simulink library "lddc_lib"  (Simulink 8.7)
settings: Solver=ode45  StartTime=0.0  StopTime=10.0  RelTol=1e-3
undefined symbols (not defined in the file): DDC_LINEUP_param, display, value
libraries: DSPBAPrim x9, DSPBAFilters x6, DSPBABase x6
settings Model: Creator=bigcat  LastModifiedBy=5g

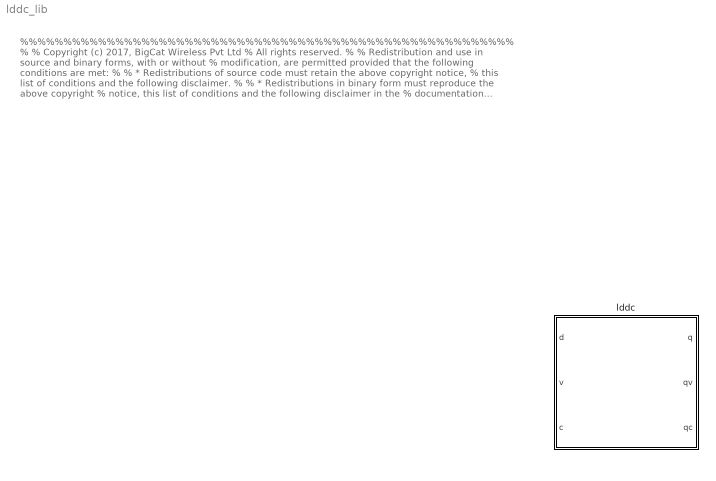
== system lddc_lib ==
  note: %%%%%%%%%%%%%%%%%%%%%%%%%%%%%%%%%%%%%%%%%%%%%%%%%%%%%%%%%
      |  %
      |  % Copyright (c) 2017, BigCat Wireless Pvt Ltd
      |  % All rights reserved.
      |  %
      |  % Redistribution and use in source and binary forms, with or without
      |  % modification, are permitted provided that the following conditions are met:
      |  %
      |  %     * Redistributions of source code must retain the above copyright notice,
      |  %       this list of conditions and the following disclaimer.
      |  %
      |  %     * Redistributions in binary form must reproduce the above copyright
      |  %       notice, this list of conditions and the following disclaimer in the
      |  %       documentation and/or other materials provided with the distribution.
      |  %
      |  %     * Neither the name of the copyright holder nor the names of its contributors
      |  %       may be used to endorse or promote products derived from this software
      |  %       without specific prior written permission.
      |  %
      |  %
      |  %
      |  % THIS SOFTWARE IS PROVIDED BY THE COPYRIGHT HOLDERS AND CONTRIBUTORS "AS IS"
      |  % AND ANY EXPRESS OR IMPLIED WARRANTIES, INCLUDING, BUT NOT LIMITED TO, THE
      |  % IMPLIED WARRANTIES OF MERCHANTABILITY AND FITNESS FOR A PARTICULAR PURPOSE ARE
      |  % DISCLAIMED. IN NO EVENT SHALL THE COPYRIGHT HOLDER OR CONTRIBUTORS BE LIABLE
      |  % FOR ANY DIRECT, INDIRECT, INCIDENTAL, SPECIAL, EXEMPLARY, OR CONSEQUENTIAL
      |  % DAMAGES (INCLUDING, BUT NOT LIMITED TO, PROCUREMENT OF SUBSTITUTE GOODS OR
      |  % SERVICES; LOSS OF USE, DATA, OR PROFITS; OR BUSINESS INTERRUPTION) HOWEVER
      |  % CAUSED AND ON ANY THEORY OF LIABILITY, WHETHER IN CONTRACT, STRICT LIABILITY,
      |  % OR TORT (INCLUDING NEGLIGENCE OR OTHERWISE) ARISING IN ANY WAY OUT OF THE USE
      |  % OF THIS SOFTWARE, EVEN IF ADVISED OF THE POSSIBILITY OF SUCH DAMAGE.
      |  %
      |   %%%%%%%%%%%%%%%%%%%%%%%%%%%%%%%%%%%%%%%%%%%%%%%%%%%%%
  lddc : Subsystem  mask{HB5_filter_SampleRate=DDC_LINEUP_param.HB_filter5.SampleRate, HB5_filter_Decimation=DDC_LINEUP_param.HB_filter5.Decimation, HB5_filter_ChanCount=DDC_LINEUP_param.HB_filter5.ChanCount, HB5_filter_coeffs=DDC_LINEUP_param.HB_filt5.coeffs(1,:), HB5_filter_base_addr=DDC_LINEUP_param.HB_filter5.base_addr, HB4_filter_SampleRate=DDC_LINEUP_param.HB_filter4.SampleRate, HB4_filter_Decimation=DDC_LINEUP_param.HB_filter4.Decimation, HB4_filter_ChanCount=DDC_LINEUP_param.HB_filter4.ChanCount, HB4_filter_coeffs=DDC_LINEUP_param.HB_filt4.coeffs(1,:), HB4_filter_base_addr=DDC_LINEUP_param.HB_filter4.base_addr, CH_filter_SampleRate=DDC_LINEUP_param.CH_filter.SampleRate, CH_filter_ChanCount=DDC_LINEUP_param.CH_filter.ChanCount, CH_filter_coeffs=DDC_LINEUP_param.chan_filter.coeffs(1,:), CH_filter_base_addr=DDC_LINEUP_param.CH_filter.base_addr, output_word_length=DDC_LINEUP_param.output_word_length, output_fraction_length=DDC_LINEUP_param.output_fraction_length, Pipeline_stages=2, Clock_Margin=DDC_LINEUP_param.ClockMargin}
      mask Display:
      | disp('LDDC');
      | port_label('input',1,'d');
      | port_label('input',2,'v');
      | port_label('input',3,'c');
      | port_label('output',1,'q');
      | port_label('output',2,'q_v');
      | port_label('output',3,'q_c');

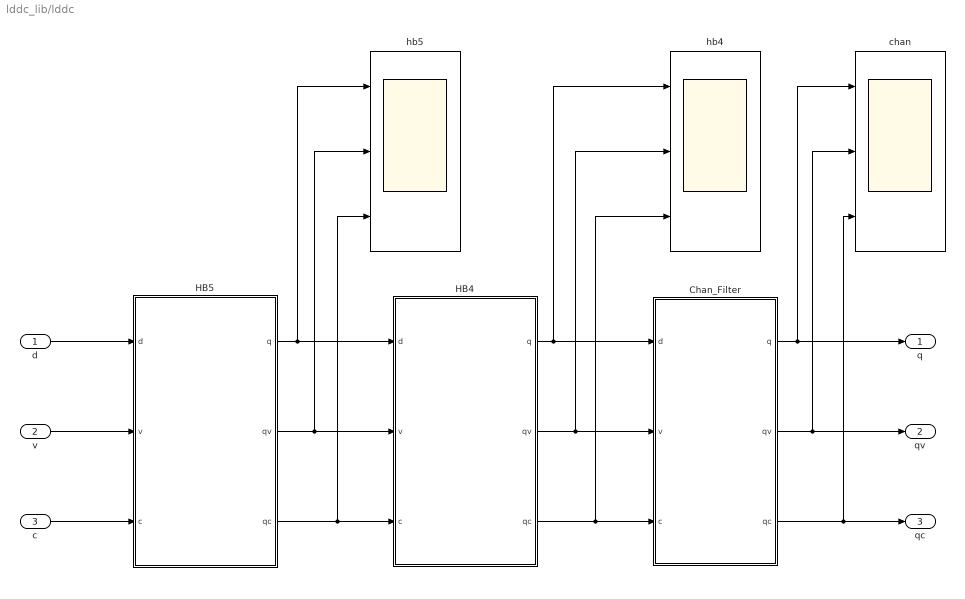
== system lddc_lib/lddc ==
  d : Inport
  v : Inport  Port=2
  c : Inport  Port=3
  Chan_Filter : Subsystem
  HB4 : Subsystem
  HB5 : Subsystem
  chan : Scope  NumInputPorts=3
  hb4 : Scope  NumInputPorts=3
  hb5 : Scope  NumInputPorts=3
  q : Outport
  qv : Outport  Port=2
  qc : Outport  Port=3
  wires:
  HB4/3(qc) -> hb4/3, Chan_Filter/3(c)
  HB4/2(qv) -> hb4/2, Chan_Filter/2(v)
  HB4/1(q) -> hb4/1, Chan_Filter/1(d)
  HB5/3(qc) -> hb5/3, HB4/3(c)
  HB5/2(qv) -> hb5/2, HB4/2(v)
  HB5/1(q) -> hb5/1, HB4/1(d)
  d/1 -> HB5/1(d)
  v/1 -> HB5/2(v)
  c/1 -> HB5/3(c)
  Chan_Filter/1(q) -> chan/1, q/1
  Chan_Filter/2(qv) -> chan/2, qv/1
  Chan_Filter/3(qc) -> chan/3, qc/1

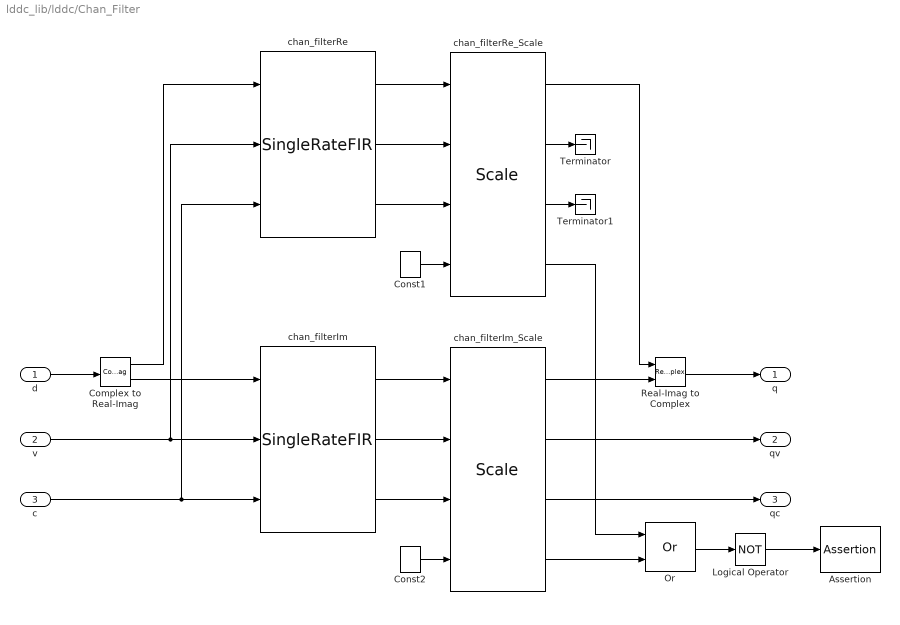
== system lddc_lib/lddc/Chan_Filter ==
  d : Inport
  v : Inport  Port=2
  c : Inport  Port=3
  Assertion : Assertion  Enabled=off  AssertionFailFcn=display('Simulation stopped, because an over/underflow was detected in LDDC/HB5')
  Complex to Real-Imag : ComplexToRealImag
  Const1 : DSPBAPrim/Const  primtype=const  nInputs=0  nOutputs=1  omode=Inherit via internal rule  otype=sfix(16)  scale=2^-15  rndmethod=Unbiased  factor=1  satmethod=Symmetric  shift_vec=[0 1 2 -1]  value=0  inPortNames=['+'; '+';]  outPortNames=[' ']  dspbaimage=dspba_prim.jpg  text=fprintf('%s', num2str(value));  style=Optimised  visibilities=8 + 1024  floatPrecision=float32_m23  version=20120820
  Const2 : DSPBAPrim/Const  primtype=const  nInputs=0  nOutputs=1  omode=Inherit via internal rule  otype=sfix(16)  scale=2^-15  rndmethod=Unbiased  factor=1  satmethod=Symmetric  shift_vec=[0 1 2 -1]  value=0  inPortNames=['+'; '+';]  outPortNames=[' ']  dspbaimage=dspba_prim.jpg  text=fprintf('%s', num2str(value));  style=Optimised  visibilities=8 + 1024  floatPrecision=float32_m23  version=20120820
  Logical Operator : Logic  Operator=NOT  AllPortsSameDT=off  OutDataTypeStr=boolean
  Or : DSPBAPrim/Or  primtype=or  nInputs=2  nOutputs=1  omode=Inherit via internal rule  otype=sfix(16)  scale=2^-15  rndmethod=Unbiased  factor=1  satmethod=Symmetric  shift_vec=[0 1 2 -1]  value=0  inPortNames=[' '; ' '; ' '; ' '; ' '; ' '; ' '; ' '; ' '; ' '; ' '; ' '; ' '; ' '; ' '; ' '; ]  outPortNames=[' ']  dspbaimage=dspba_prim.jpg  text=fprintf('|');  style=Optimised  visibilities=8+2  version=20090407
  Real-Imag to Complex : RealImagToComplex
  Terminator : Terminator
  Terminator1 : Terminator
  chan_filterIm : DSPBAFilters/SingleRateFIR  nInputRate=CH_filter_SampleRate  nchan=CH_filter_ChanCount  symmetry=Symmetrical  coef=fi(CH_filter_coeffs,1,16,15)  addr=CH_filter_base_addr+64  rwmode=Read/Write  nband=Use All Taps  latency=4  exposebus=off  version=20090407  recon=off  MM=[0,1,2,3,4,5,6,7,8,9,10,11,12,13,14,15,16,17,18,19]
  chan_filterIm_Scale : DSPBABase/Scale  otype=sfix(output_word_length)  scale=2^-output_fraction_length  rndmethod=Truncate  factor=1  satmethod=Symmetric  shift_vec=0  latency=4  wideSimulation=off  version=20130807
  chan_filterRe : DSPBAFilters/SingleRateFIR  nInputRate=CH_filter_SampleRate  nchan=CH_filter_ChanCount  symmetry=Symmetrical  coef=fi(CH_filter_coeffs,1,16,15)  addr=CH_filter_base_addr  rwmode=Read/Write  nband=Use All Taps  latency=4  exposebus=off  version=20090407  recon=off  MM=[0,1,2,3,4,5,6,7,8,9,10,11,12,13,14,15,16,17,18,19]
  chan_filterRe_Scale : DSPBABase/Scale  otype=sfix(output_word_length)  scale=2^-output_fraction_length  rndmethod=Truncate  factor=1  satmethod=Symmetric  shift_vec=0  latency=4  wideSimulation=off  version=20130807
  q : Outport
  qv : Outport  Port=2
  qc : Outport  Port=3
  wires:
  v/1 -> chan_filterIm/2, chan_filterRe/2
  Or/1 -> Logical Operator/1
  Logical Operator/1 -> Assertion/1
  Real-Imag to Complex/1 -> q/1
  chan_filterIm_Scale/1 -> Real-Imag to Complex/2
  chan_filterRe_Scale/1 -> Real-Imag to Complex/1
  chan_filterRe_Scale/4 -> Or/1
  chan_filterIm_Scale/4 -> Or/2
  Complex to Real-Imag/1 -> chan_filterRe/1
  Complex to Real-Imag/2 -> chan_filterIm/1
  d/1 -> Complex to Real-Imag/1
  chan_filterRe/2 -> chan_filterRe_Scale/2
  chan_filterRe/3 -> chan_filterRe_Scale/3
  Const1/1 -> chan_filterRe_Scale/4
  chan_filterRe/1 -> chan_filterRe_Scale/1
  chan_filterIm/2 -> chan_filterIm_Scale/2
  chan_filterIm/3 -> chan_filterIm_Scale/3
  chan_filterIm_Scale/2 -> qv/1
  Const2/1 -> chan_filterIm_Scale/4
  chan_filterIm_Scale/3 -> qc/1
  chan_filterIm/1 -> chan_filterIm_Scale/1
  c/1 -> chan_filterIm/3, chan_filterRe/3
  chan_filterRe_Scale/2 -> Terminator/1
  chan_filterRe_Scale/3 -> Terminator1/1

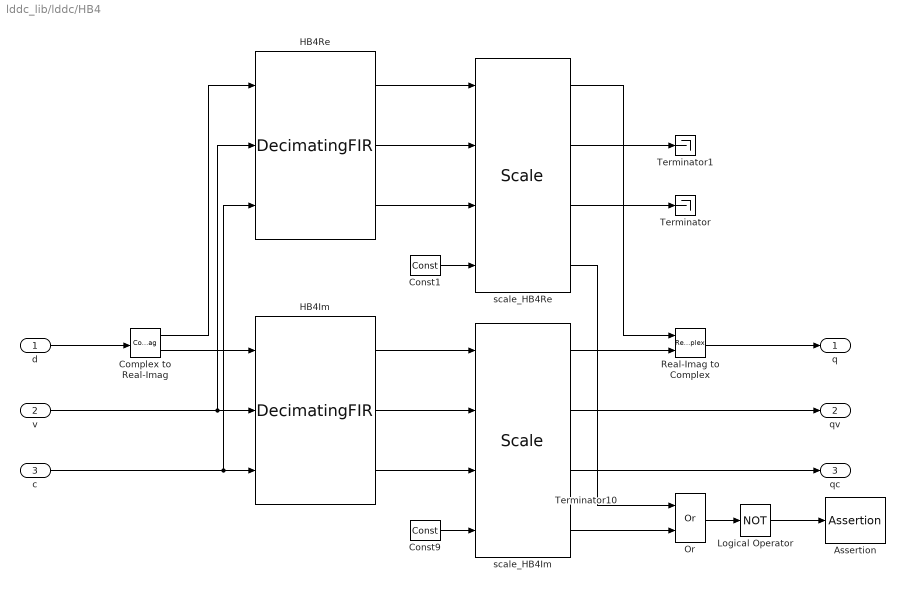
== system lddc_lib/lddc/HB4 ==
  d : Inport
  v : Inport  Port=2
  c : Inport  Port=3
  Assertion : Assertion  Enabled=off  AssertionFailFcn=display('Simulation stopped, because an over/underflow was detected in LDDC/HB4')
  Complex to Real-Imag : ComplexToRealImag
  Const1 : DSPBAPrim/Const  primtype=const  nInputs=0  nOutputs=1  omode=Inherit via internal rule  otype=sfix(16)  scale=2^-15  rndmethod=Unbiased  factor=1  satmethod=Symmetric  shift_vec=[0 1 2 -1]  value=0  inPortNames=['+'; '+';]  outPortNames=[' ']  dspbaimage=dspba_prim.jpg  text=fprintf('%s', num2str(value));  style=Optimised  visibilities=8 + 1024  floatPrecision=float32_m23  version=20120820
  Const9 : DSPBAPrim/Const  primtype=const  nInputs=0  nOutputs=1  omode=Inherit via internal rule  otype=sfix(16)  scale=2^-15  rndmethod=Unbiased  factor=1  satmethod=Symmetric  shift_vec=[0 1 2 -1]  value=0  inPortNames=['+'; '+';]  outPortNames=[' ']  dspbaimage=dspba_prim.jpg  text=fprintf('%s', num2str(value));  style=Optimised  visibilities=8 + 1024  floatPrecision=float32_m23  version=20120820
  HB4Im : DSPBAFilters/DecimatingFIR  nInputRate=HB4_filter_SampleRate  decim=HB4_filter_Decimation  nchan=HB4_filter_ChanCount  symmetry=Symmetrical  coef=HB4_filter_coeffs  addr=HB4_filter_base_addr  rwmode=Constant  nband=Half Band  exposebus=off  latency=23  version=20090407  recon=off  MM=[0,1,2,3,4,5,6,7,8,9,10,11,12,13,14,15]
  HB4Re : DSPBAFilters/DecimatingFIR  nInputRate=HB4_filter_SampleRate  decim=HB4_filter_Decimation  nchan=HB4_filter_ChanCount  symmetry=Symmetrical  coef=HB4_filter_coeffs  addr=HB4_filter_base_addr  rwmode=Constant  nband=Half Band  exposebus=off  latency=23  version=20090407  recon=off  MM=[0,1,2,3,4,5,6,7,8,9,10,11,12,13,14,15]
  Logical Operator : Logic  Operator=NOT  AllPortsSameDT=off  OutDataTypeStr=boolean
  Or : DSPBAPrim/Or  primtype=or  nInputs=2  nOutputs=1  omode=Inherit via internal rule  otype=sfix(16)  scale=2^-15  rndmethod=Unbiased  factor=1  satmethod=Symmetric  shift_vec=[0 1 2 -1]  value=0  inPortNames=[' '; ' '; ' '; ' '; ' '; ' '; ' '; ' '; ' '; ' '; ' '; ' '; ' '; ' '; ' '; ' '; ]  outPortNames=[' ']  dspbaimage=dspba_prim.jpg  text=fprintf('|');  style=Optimised  visibilities=8+2  version=20090407
  Real-Imag to Complex : RealImagToComplex
  Terminator : Terminator
  Terminator1 : Terminator
  Terminator10 : Terminator
  scale_HB4Im : DSPBABase/Scale  otype=sfix(output_word_length)  scale=2^-output_fraction_length  rndmethod=Truncate  factor=1  satmethod=Symmetric  shift_vec=0  latency=4  wideSimulation=off  version=20130807
  scale_HB4Re : DSPBABase/Scale  otype=sfix(output_word_length)  scale=2^-output_fraction_length  rndmethod=Truncate  factor=1  satmethod=Symmetric  shift_vec=0  latency=4  wideSimulation=off  version=20130807
  q : Outport
  qv : Outport  Port=2
  qc : Outport  Port=3
  wires:
  v/1 -> HB4Im/2, HB4Re/2
  Or/1 -> Logical Operator/1
  Logical Operator/1 -> Assertion/1
  scale_HB4Im/1 -> Real-Imag to Complex/2
  scale_HB4Re/4 -> Or/1
  scale_HB4Re/1 -> Real-Imag to Complex/1
  Complex to Real-Imag/2 -> HB4Im/1
  Complex to Real-Imag/1 -> HB4Re/1
  Real-Imag to Complex/1 -> q/1
  scale_HB4Im/4 -> Or/2
  d/1 -> Complex to Real-Imag/1
  HB4Re/3 -> scale_HB4Re/3
  HB4Re/1 -> scale_HB4Re/1
  HB4Re/2 -> scale_HB4Re/2
  Const1/1 -> scale_HB4Re/4
  HB4Im/3 -> scale_HB4Im/3
  HB4Im/1 -> scale_HB4Im/1
  HB4Im/2 -> scale_HB4Im/2
  Const9/1 -> scale_HB4Im/4
  c/1 -> HB4Im/3, HB4Re/3
  scale_HB4Im/3 -> qc/1
  scale_HB4Im/2 -> qv/1
  scale_HB4Re/3 -> Terminator/1
  scale_HB4Re/2 -> Terminator1/1

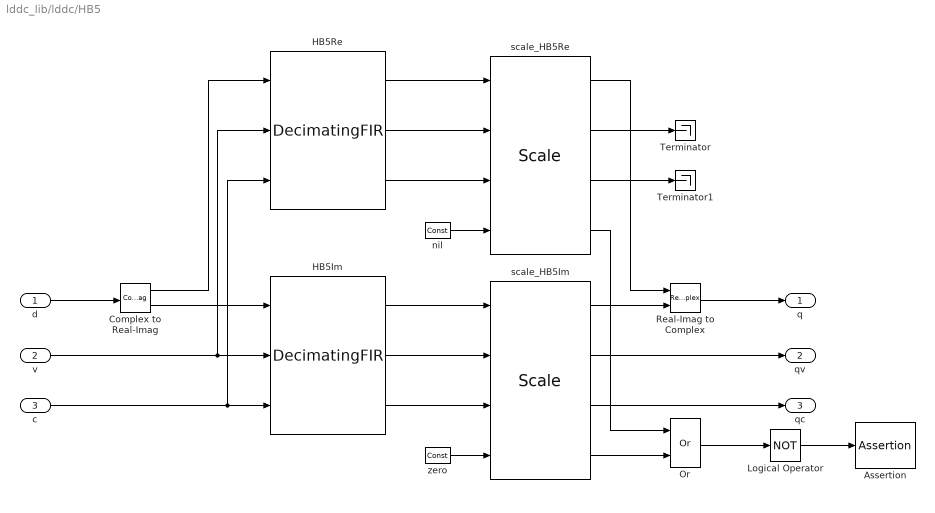
== system lddc_lib/lddc/HB5 ==
  d : Inport
  v : Inport  Port=2
  c : Inport  Port=3
  Assertion : Assertion  Enabled=off  AssertionFailFcn=display('Simulation stopped, because an over/underflow was detected in LDDC/HB5')
  Complex to Real-Imag : ComplexToRealImag
  HB5Im : DSPBAFilters/DecimatingFIR  nInputRate=HB5_filter_SampleRate  decim=HB5_filter_Decimation  nchan=HB5_filter_ChanCount  symmetry=Symmetrical  coef=HB5_filter_coeffs  addr=HB5_filter_base_addr  rwmode=Constant  nband=Half Band  exposebus=off  latency=19  version=20090407  recon=off  MM=[0,1,2,3,4,5,6,7,8,9,10,11,12,13,14,15]
  HB5Re : DSPBAFilters/DecimatingFIR  nInputRate=HB5_filter_SampleRate  decim=HB5_filter_Decimation  nchan=HB5_filter_ChanCount  symmetry=Symmetrical  coef=HB5_filter_coeffs  addr=HB5_filter_base_addr  rwmode=Constant  nband=Half Band  exposebus=off  latency=19  version=20090407  recon=off  MM=[0,1,2,3,4,5,6,7,8,9,10,11,12,13,14,15]
  Logical Operator : Logic  Operator=NOT  AllPortsSameDT=off  OutDataTypeStr=boolean
  Or : DSPBAPrim/Or  primtype=or  nInputs=2  nOutputs=1  omode=Inherit via internal rule  otype=sfix(16)  scale=2^-15  rndmethod=Unbiased  factor=1  satmethod=Symmetric  shift_vec=[0 1 2 -1]  value=0  inPortNames=[' '; ' '; ' '; ' '; ' '; ' '; ' '; ' '; ' '; ' '; ' '; ' '; ' '; ' '; ' '; ' '; ]  outPortNames=[' ']  dspbaimage=dspba_prim.jpg  text=fprintf('|');  style=Optimised  visibilities=8+2  version=20090407
  Real-Imag to Complex : RealImagToComplex
  Terminator : Terminator
  Terminator1 : Terminator
  nil : DSPBAPrim/Const  primtype=const  nInputs=0  nOutputs=1  omode=Inherit via internal rule  otype=sfix(16)  scale=2^-15  rndmethod=Unbiased  factor=1  satmethod=Symmetric  shift_vec=[0 1 2 -1]  value=0  inPortNames=['+'; '+';]  outPortNames=[' ']  dspbaimage=dspba_prim.jpg  text=fprintf('%s', num2str(value));  style=Optimised  visibilities=8 + 1024  floatPrecision=float32_m23  version=20120820
  scale_HB5Im : DSPBABase/Scale  otype=sfix(output_word_length)  scale=2^-output_fraction_length  rndmethod=Truncate  factor=1  satmethod=Symmetric  shift_vec=0  latency=4  wideSimulation=off  version=20130807
  scale_HB5Re : DSPBABase/Scale  otype=sfix(output_word_length)  scale=2^-output_fraction_length  rndmethod=Truncate  factor=1  satmethod=Symmetric  shift_vec=0  latency=4  wideSimulation=off  version=20130807
  zero : DSPBAPrim/Const  primtype=const  nInputs=0  nOutputs=1  omode=Inherit via internal rule  otype=sfix(16)  scale=2^-15  rndmethod=Unbiased  factor=1  satmethod=Symmetric  shift_vec=[0 1 2 -1]  value=0  inPortNames=['+'; '+';]  outPortNames=[' ']  dspbaimage=dspba_prim.jpg  text=fprintf('%s', num2str(value));  style=Optimised  visibilities=8 + 1024  floatPrecision=float32_m23  version=20120820
  q : Outport
  qv : Outport  Port=2
  qc : Outport  Port=3
  wires:
  v/1 -> HB5Im/2, HB5Re/2
  Logical Operator/1 -> Assertion/1
  Or/1 -> Logical Operator/1
  Complex to Real-Imag/1 -> HB5Re/1
  scale_HB5Re/4 -> Or/1
  scale_HB5Im/4 -> Or/2
  scale_HB5Re/1 -> Real-Imag to Complex/1
  scale_HB5Im/1 -> Real-Imag to Complex/2
  Real-Imag to Complex/1 -> q/1
  Complex to Real-Imag/2 -> HB5Im/1
  d/1 -> Complex to Real-Imag/1
  HB5Re/3 -> scale_HB5Re/3
  HB5Re/2 -> scale_HB5Re/2
  nil/1 -> scale_HB5Re/4
  HB5Re/1 -> scale_HB5Re/1
  HB5Im/3 -> scale_HB5Im/3
  HB5Im/2 -> scale_HB5Im/2
  zero/1 -> scale_HB5Im/4
  HB5Im/1 -> scale_HB5Im/1
  scale_HB5Im/2 -> qv/1
  scale_HB5Im/3 -> qc/1
  c/1 -> HB5Im/3, HB5Re/3
  scale_HB5Re/2 -> Terminator/1
  scale_HB5Re/3 -> Terminator1/1
